simulink model "AM_superheterodyne_image_2020"  (R2020b)
settings: Solver=ode45  StartTime=0.0  StopTime=12e-3  FixedStep=1/32000  RelTol=1e-3  EnableMultiTasking=on
PreLoadFcn:
  | fRF=560000;
  | Df=0;
  | fIF=455000;
  | W=10000;
  | Ts=1/3.25e6;
values from neighbouring files (symbols this model uses):
  seed = input('Enter your student ID: ')    [DSBAMsignals.m]    (also in DSBAMsignals_rand.m; DSB_SC_sinusoidals.m)
libraries: dsparch4 x5, simulink x1
settings Model: Creator=Research  LastModifiedBy=14083
settings DataIOCC: LimitDataPoints=on  SaveFormat=Array  SignalLoggingSaveFormat=ModelDataLogs  ReturnWorkspaceOutputs=off
settings OptimizationCC: ExpressionDepthLimit=2147483647  InitFltsAndDblsToZero=on  LifeSpan=inf
settings DebuggingCC: SaveWithParameterizedLinksMsg=none  UnderspecifiedInitializationDetection=Classic  MergeDetectMultiDrivingBlocksExec=none  SignalResolutionControl=TryResolveAllWithWarning  SolverPrmCheckMsg=warning  MultiTaskDSMMsg=warning  MultiTaskCondExecSysMsg=none  FcnCallInpInsideContextMsg=warning  StateNameClashWarn=warning  SFUnexpectedBacktrackingDiag=warning  SFNoUnconditionalDefaultTransitionDiag=warning  SFExecutionAtInitializationDiag=none  ArithmeticOperatorsInVariantConditions=warning
settings HardwareCC: ProdBitPerPointer=32  ProdBitPerSizeT=32  ProdBitPerPtrDiffT=32  ProdLargestAtomicFloat=None  ProdIntDivRoundTo=Undefined  ProdEndianess=Unspecified  ProdWordSize=32  ProdHWDeviceType=32-bit Generic
settings ModelReferenceCC: PropagateSignalLabelsOutOfModel=off
settings SFSimCC: SimUseLocalCustomCode=off  CustomCodeUndefinedFunction=UseInterfaceOnly
settings RTWCC: RTWUseLocalCustomCode=off
settings CodeAppCC: StateflowObjectComments=on
settings GRTTargetCC: TargetFcnLib=ansi_tfl_tmw.mat  TargetLangStandard=C89/C90 (ANSI)  CombineOutputUpdateFcns=off  GRTInterface=on
settings ConfigComp: CovMetricSettings=dw  CovSaveCumulativeToWorkspaceVar=on  CovSaveSingleToWorkspaceVar=on  CovExternalEMLEnable=off

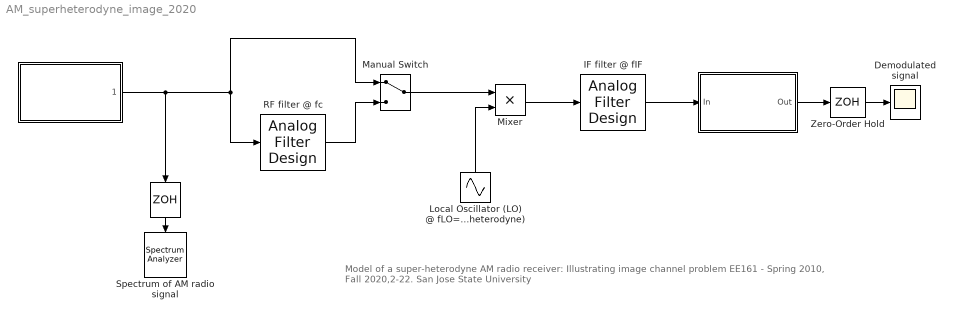
== system AM_superheterodyne_image_2020 ==
  note: Model of a super-heterodyne AM radio receiver:
      | Illustrating image channel problem
      | EE161 - Spring 2010, Fall 2020,2-22. San Jose State University
  " " : Subsystem  TreatAsAtomicUnit=on
      mask Display: disp('Detected\nAM signals')
  "  " : ZeroOrderHold  SampleTime=Ts
  "    " : Subsystem  TreatAsAtomicUnit=on
      mask Display: disp('Envelope\nDetector')
  "  Local Oscillator (LO) @ fLO=fc+fIF (Superheterodyne)" : Sin  Frequency=2*pi*(fRF+fIF+Df)  SampleTime=Ts
  " RF filter @ fc" : dsparch4/Analog Filter Design  method=Butterworth  filttype=Bandpass  N=4  Wlo=2*pi*(fRF-7*W)  Whi=2*pi*(fRF+7*W)  Rp=2  Rs=40
  Demodulated signal : Scope
  IF filter @ fIF : dsparch4/Analog Filter Design  method=Butterworth  filttype=Bandpass  N=4  Wlo=2*pi*(fIF-W)  Whi=2*pi*(fIF+W)  Rp=2  Rs=40
  Manual Switch : ManualSwitch
  Mixer : Product  RndMeth=Zero
  Spectrum of AM radio signal : SpectrumAnalyzer
  Zero-Order Hold : ZeroOrderHold  SampleTime=2e-7
  wires:
  Mixer/1 -> IF filter @ fIF/1
  "  "/1 -> Spectrum of AM radio signal/1
  IF filter @ fIF/1 -> "    "/1(In)
  Zero-Order Hold/1 -> Demodulated signal/1
  " "/1("    ") -> " RF filter @ fc"/1, Manual Switch/1, "  "/1
  "    "/1(Out) -> Zero-Order Hold/1
  Manual Switch/1 -> Mixer/1
  " RF filter @ fc"/1 -> Manual Switch/2
  "  Local Oscillator (LO) @ fLO=fc+fIF (Superheterodyne)"/1 -> Mixer/2

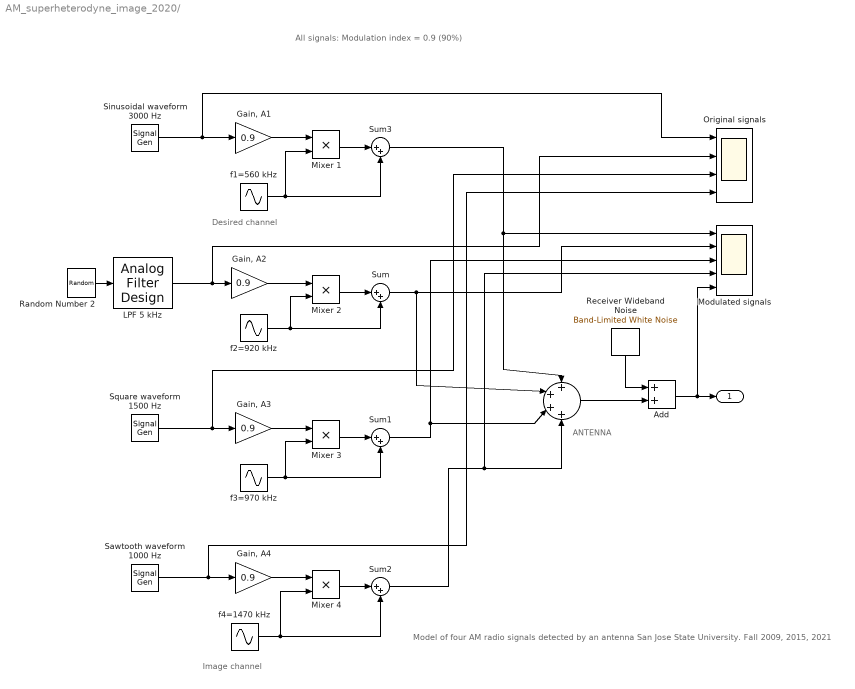
== system AM_superheterodyne_image_2020/  ==
  note: All signals: Modulation index = 0.9 (90%)
  note: Model of four AM radio signals detected by an antenna
      | San Jose State University. Fall 2009, 2015, 2021
  note: ANTENNA
  note: Desired channel
  note: Image channel
  " " : Sum  Inputs=++++
  " Receiver Wideband Noise" : simulink/Sources/Band-Limited White Noise  Cov=1e-8  Ts=Ts  seed=seed+147813
  Add : Sum
  "Gain, A1" : Gain  Gain=0.9
  "Gain, A2 " : Gain  Gain=0.9
  "Gain, A3 " : Gain  Gain=0.9
  "Gain, A4 " : Gain  Gain=0.9
  LPF 5 kHz : dsparch4/Analog Filter Design  method=Butterworth  filttype=Lowpass  N=6  Wlo=2*pi*5000  Whi=2*pi*110  Rp=1  Rs=40
  Mixer {1..4} (4 alike) : Product  RndMeth=Zero
  Modulated signals : Scope  NumInputPorts=5
  Original signals : Scope  NumInputPorts=4
  Random Number 2 : UniformRandomNumber  Seed=seed  SampleTime=1e-4
  Sawtooth waveform 1000 Hz : SignalGenerator  WaveForm=sawtooth  Frequency=888
  Sinusoidal waveform 3000 Hz : SignalGenerator  Frequency=3000
  Square waveform 1500 Hz : SignalGenerator  WaveForm=square  Frequency=1500
  Sum{,1..3} (4 alike) : Sum  Inputs=|++
  f1=560 kHz : Sin  Frequency=2*pi*560000  SampleTime=Ts
  f2=920 kHz : Sin  Frequency=2*pi*920000  SampleTime=Ts
  f3=970 kHz : Sin  Frequency=2*pi*970000  SampleTime=Ts
  f4=1470 kHz : Sin  Frequency=2*pi*1470000  SampleTime=Ts
  "    " : Outport
  wires:
  LPF 5 kHz/1 -> Original signals/2, "Gain, A2 "/1
  f2=920 kHz/1 -> Mixer 2/2, Sum/2
  Square waveform 1500 Hz/1 -> Original signals/3, "Gain, A3 "/1
  f3=970 kHz/1 -> Mixer 3/2, Sum1/2
  Sawtooth waveform 1000 Hz/1 -> Original signals/4, "Gain, A4 "/1
  f4=1470 kHz/1 -> Mixer 4/2, Sum2/2
  Mixer 2/1 -> Sum/1
  Mixer 3/1 -> Sum1/1
  Mixer 4/1 -> Sum2/1
  Sum/1 -> Modulated signals/2, " "/2
  Sum1/1 -> " "/3, Modulated signals/3
  Sum2/1 -> " "/4, Modulated signals/4
  Sinusoidal waveform 3000 Hz/1 -> Original signals/1, "Gain, A1"/1
  Mixer 1/1 -> Sum3/1
  Sum3/1 -> " "/1, Modulated signals/1
  " Receiver Wideband Noise"/1 -> Add/1
  " "/1 -> Add/2
  Add/1 -> "    "/1, Modulated signals/5
  Random Number 2/1 -> LPF 5 kHz/1
  "Gain, A1"/1 -> Mixer 1/1
  f1=560 kHz/1 -> Mixer 1/2, Sum3/2
  "Gain, A2 "/1 -> Mixer 2/1
  "Gain, A3 "/1 -> Mixer 3/1
  "Gain, A4 "/1 -> Mixer 4/1

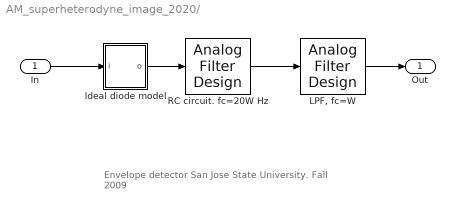
== system AM_superheterodyne_image_2020/     ==
  note: Envelope detector
      | San Jose State University. Fall 2009
  In : Inport
  Ideal diode model : Subsystem  TreatAsAtomicUnit=on
  "LPF, fc=W" : dsparch4/Analog Filter Design  method=Butterworth  filttype=Lowpass  N=2  Wlo=2*pi*W  Whi=2*pi*110  Rp=2  Rs=60
  RC circuit. fc=20W Hz : dsparch4/Analog Filter Design  method=Butterworth  filttype=Lowpass  N=1  Wlo=40*pi*W  Whi=2*pi*110  Rp=2  Rs=60
  Out : Outport
  wires:
  Ideal diode model/1(o) -> RC circuit. fc=20W Hz/1
  In/1 -> Ideal diode model/1(i)
  RC circuit. fc=20W Hz/1 -> "LPF, fc=W"/1
  "LPF, fc=W"/1 -> Out/1

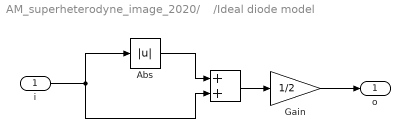
== system AM_superheterodyne_image_2020/    /Ideal diode model ==
  i : Inport
  " " : Sum
  Abs : Abs
  Gain : Gain  Gain=1/2
  o : Outport
  wires:
  i/1 -> Abs/1, " "/2
  Abs/1 -> " "/1
  " "/1 -> Gain/1
  Gain/1 -> o/1
